simulink library "walk_left_Gait"  (R2024a)
settings: Solver=VariableStepAuto  StartTime=0.0  StopTime=10.0  RelTol=1e-3
undefined symbols (not defined in the file): Lower_limbs, Upper_limbs
libraries: Plane_Movement_walk_left x4
settings Model: Creator=renre  LastModifiedBy=leona

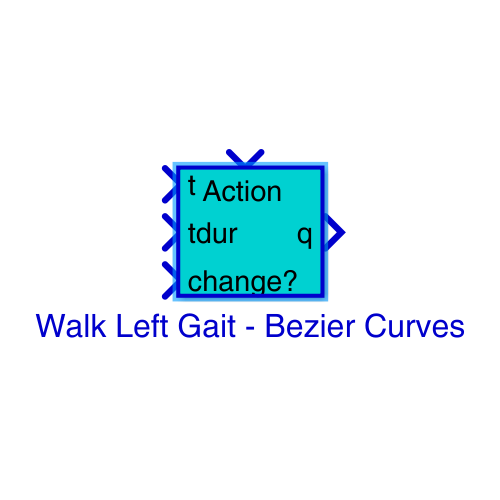
[thumbnail: Simulink's stored preview of the top-level diagram]
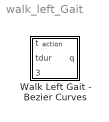
== system walk_left_Gait ==
  Walk Left Gait - Bezier Curves : Subsystem  mask{P0x=-0.02, P0z=-0.08, P1x=-0.035, P1z=-0.06, P2x=0.01, P2z=-0.075, P3x=0.02, P3z=-0.08}
      mask prompts: P0x "Bezier-Point 0 - X"; P0z "Bezier-Point 0 - Z"; P1x "Bezier-Point 1 - X"; P1z "Bezier-Point 1- Z"; P2x "Bezier-Point 2 - X"; P2z "Bezier-Point 2 - Z"; P3x "Bezier-Point 3 - X"; P3z "Bezier-Point 3- Z"

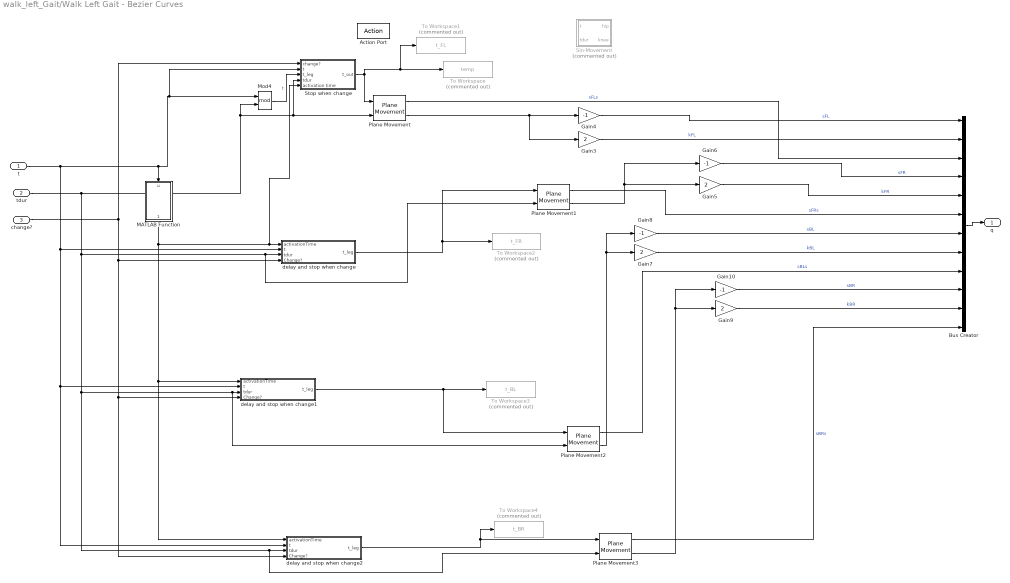
== system walk_left_Gait/Walk Left Gait - Bezier Curves ==
  t : Inport
  tdur : Inport  Port=2
  change? : Inport  Port=3
  Action Port : ActionPort  InitializeStates=reset
  Bus Creator : BusCreator  Inputs=12
  Gain{4,6,8,10} (4 alike) : Gain  Gain=-1
  Gain{3,5,7,9} (4 alike) : Gain  Gain=2
  MATLAB Function : MATLAB Function  TreatAsAtomicUnit=on
  Mod4 : Math  Operator=mod
  Plane Movement{,1..3} (4 alike) : Plane_Movement_walk_left/Plane Movement  SystemSampleTime=-1  VariantActivationTime=update diagram  AllowFlexibleInterface=on  Latency=0  AutoFrameSizeCalculation=off
  Sin-Movement : Subsystem  Commented=on
  Stop when change : Subsystem
  To Workspace : ToWorkspace  Commented=on  VariableName=temp  SaveFormat=Structure With Time  SampleTime=-1
  To Workspace1 : ToWorkspace  Commented=on  VariableName=t_FL  SaveFormat=Structure With Time  SampleTime=-1
  To Workspace2 : ToWorkspace  Commented=on  VariableName=t_FR  SaveFormat=Structure  SampleTime=-1
  To Workspace3 : ToWorkspace  Commented=on  VariableName=t_BL  SaveFormat=Structure  SampleTime=-1
  To Workspace4 : ToWorkspace  Commented=on  VariableName=t_BR  SaveFormat=Structure  SampleTime=-1
  delay and stop when change : Subsystem  mask{delay=0.5}
  delay and stop when change1 : Subsystem  mask{delay=0.25}
  delay and stop when change2 : Subsystem  mask{delay=0.75}
  q : Outport
  wires:
  Bus Creator/1 -> q/1
  Plane Movement/1 -> Bus Creator/3  "sFLs"
  Plane Movement1/1 -> Bus Creator/6  "sFRs"
  Plane Movement/2 -> Gain3/1, Gain4/1
  Plane Movement1/2 -> Gain6/1, Gain5/1
  Plane Movement2/2 -> Gain7/1, Gain8/1
  Plane Movement2/1 -> Bus Creator/9  "sBLs"
  Plane Movement3/2 -> Gain10/1, Gain9/1
  Plane Movement3/1 -> Bus Creator/12  "sBRs"
  Mod4/1 -> Stop when change/3(t_leg)  "t"
  Gain4/1 -> Bus Creator/1  "sFL"
  Gain5/1 -> Bus Creator/5  "kFR"
  Gain6/1 -> Bus Creator/4  "sFR"
  Gain7/1 -> Bus Creator/8  "kBL"
  Gain8/1 -> Bus Creator/7  "sBL"
  Gain9/1 -> Bus Creator/11  "kBR"
  Gain10/1 -> Bus Creator/10  "sBR"
  Gain3/1 -> Bus Creator/2  "kFL"
  Stop when change/1(t_out) -> Plane Movement/1, To Workspace1/1, To Workspace/1
  delay and stop when change2/1(t_leg) -> To Workspace4/1, Plane Movement3/1
  delay and stop when change1/1(t_leg) -> To Workspace3/1, Plane Movement2/1
  delay and stop when change/1(t_leg) -> To Workspace2/1, Plane Movement1/1
  t/1 -> delay and stop when change2/2(t), delay and stop when change1/2(t), delay and stop when change/2(t), Stop when change/2(t), Mod4/1, MATLAB Function/1(u)
  change?/1 -> delay and stop when change2/4(Change?), delay and stop when change1/4(Change?), delay and stop when change/4(Change?), Stop when change/1(change?)
  tdur/1 -> Plane Movement1/2, delay and stop when change/3(tdur), Plane Movement3/2, delay and stop when change2/3(tdur), Plane Movement2/2, delay and stop when change1/3(tdur), Stop when change/4(tdur), Plane Movement/2, Mod4/2
  MATLAB Function/1(activationTime) -> Stop when change/5(activation time), delay and stop when change/1(activationTime), delay and stop when change2/1(activationTime), delay and stop when change1/1(activationTime)

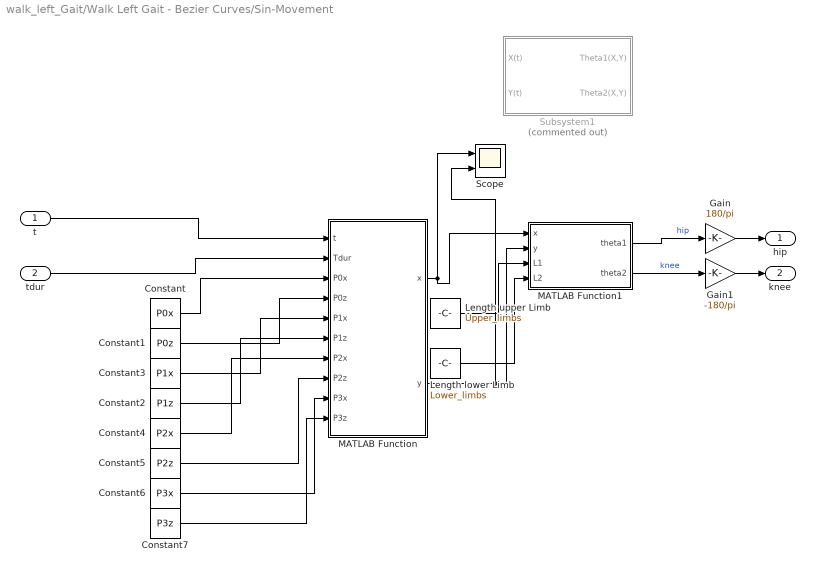
== system walk_left_Gait/Walk Left Gait - Bezier Curves/Sin-Movement ==
  t : Inport
  tdur : Inport  Port=2
  Constant : Constant  Value=P0x
  Constant1 : Constant  Value=P0z
  Constant2 : Constant  Value=P1z
  Constant3 : Constant  Value=P1x
  Constant4 : Constant  Value=P2x
  Constant5 : Constant  Value=P2z
  Constant6 : Constant  Value=P3x
  Constant7 : Constant  Value=P3z
  Gain : Gain  Gain=180/pi
  Gain1 : Gain  Gain=-180/pi
  Length lower Limb : Constant  Value=Lower_limbs
  Length upper Limb : Constant  Value=Upper_limbs
  MATLAB Function : MATLAB Function  TreatAsAtomicUnit=on
  MATLAB Function1 : MATLAB Function  TreatAsAtomicUnit=on
  Scope : Scope  NumInputPorts=2
  Subsystem1 : Subsystem  Commented=on
  hip : Outport
  knee : Outport  Port=2
  wires:
  MATLAB Function/2(y) -> MATLAB Function1/2(y), Scope/2
  MATLAB Function/1(x) -> MATLAB Function1/1(x), Scope/1
  MATLAB Function1/2(theta2) -> Gain1/1  "knee"
  tdur/1 -> MATLAB Function/2(Tdur)
  MATLAB Function1/1(theta1) -> Gain/1  "hip"
  t/1 -> MATLAB Function/1(t)
  Length upper Limb/1 -> MATLAB Function1/3(L1)
  Length lower Limb/1 -> MATLAB Function1/4(L2)
  Gain1/1 -> knee/1
  Gain/1 -> hip/1
  Constant/1 -> MATLAB Function/3(P0x)
  Constant1/1 -> MATLAB Function/4(P0z)
  Constant3/1 -> MATLAB Function/5(P1x)
  Constant2/1 -> MATLAB Function/6(P1z)
  Constant4/1 -> MATLAB Function/7(P2x)
  Constant5/1 -> MATLAB Function/8(P2z)
  Constant6/1 -> MATLAB Function/9(P3x)
  Constant7/1 -> MATLAB Function/10(P3z)

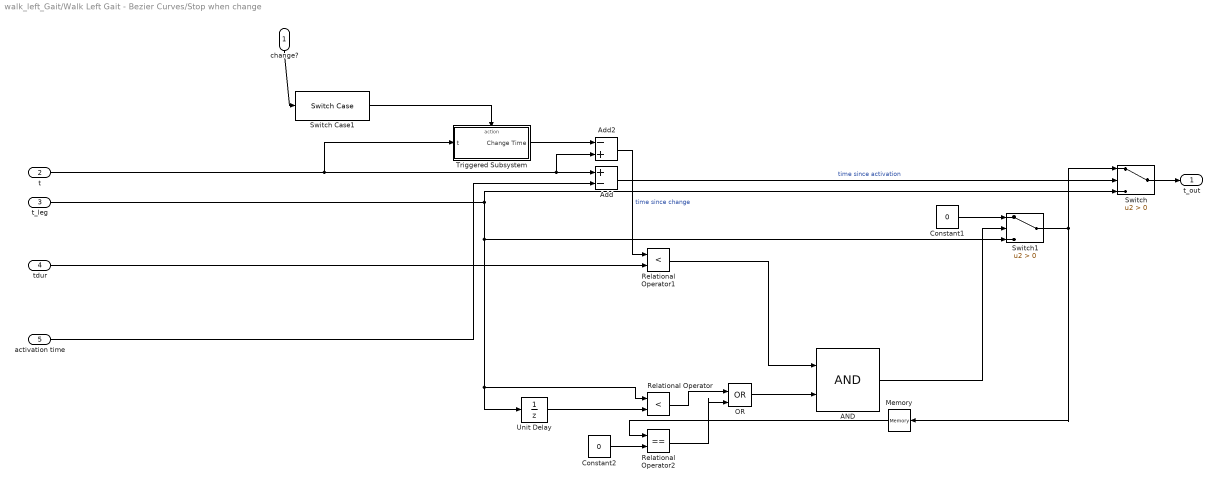
== system walk_left_Gait/Walk Left Gait - Bezier Curves/Stop when change ==
  change? : Inport
  t : Inport  Port=2
  t_leg : Inport  Port=3
  tdur : Inport  Port=4
  activation time : Inport  Port=5
  AND : Logic  IconShape=distinctive  AllPortsSameDT=off  OutDataTypeStr=boolean
  Add : Sum  Inputs=+-
  Add2 : Sum  Inputs=-+
  Constant1 : Constant  Value=0
  Constant2 : Constant  Value=0
  Memory : Memory
  OR : Logic  Operator=OR  IconShape=distinctive  AllPortsSameDT=off  OutDataTypeStr=boolean
  Relational Operator : RelationalOperator  Operator=<  OutDataTypeStr=boolean  RndMeth=Simplest  InputSameDT=off
  Relational Operator1 : RelationalOperator  Operator=<  OutDataTypeStr=boolean  RndMeth=Simplest  InputSameDT=off
  Relational Operator2 : RelationalOperator  Operator===  OutDataTypeStr=boolean  RndMeth=Simplest  InputSameDT=off
  Switch : Switch  Criteria=u2 > Threshold  SaturateOnIntegerOverflow=off  InputSameDT=off
  Switch Case1 : SwitchCase  ShowDefaultCase=off
  Switch1 : Switch  Criteria=u2 > Threshold  SaturateOnIntegerOverflow=off  InputSameDT=off
  Triggered Subsystem : Subsystem  TreatAsAtomicUnit=on
  Unit Delay : UnitDelay  SampleTime=-1  HasFrameUpgradeWarning=on
  t_out : Outport
  wires:
  t_leg/1 -> Switch1/3, Relational Operator/1, Unit Delay/1, Switch/3
  Add2/1 -> Relational Operator1/1  "time since change"
  change?/1 -> Switch Case1/1
  Switch Case1/1 -> Triggered Subsystem/Action
  AND/1 -> Switch1/2
  Unit Delay/1 -> Relational Operator/2
  Switch1/1 -> Memory/1, Switch/1
  Relational Operator1/1 -> AND/1
  Constant2/1 -> Relational Operator2/2
  Triggered Subsystem/1(Change Time) -> Add2/1
  Relational Operator/1 -> OR/1
  tdur/1 -> Relational Operator1/2
  Relational Operator2/1 -> OR/2
  OR/1 -> AND/2
  Constant1/1 -> Switch1/1
  t/1 -> Triggered Subsystem/1(t), Add2/2, Add/1
  Add/1 -> Switch/2  "time since activation"
  Switch/1 -> t_out/1
  activation time/1 -> Add/2
  Memory/1 -> Relational Operator2/1

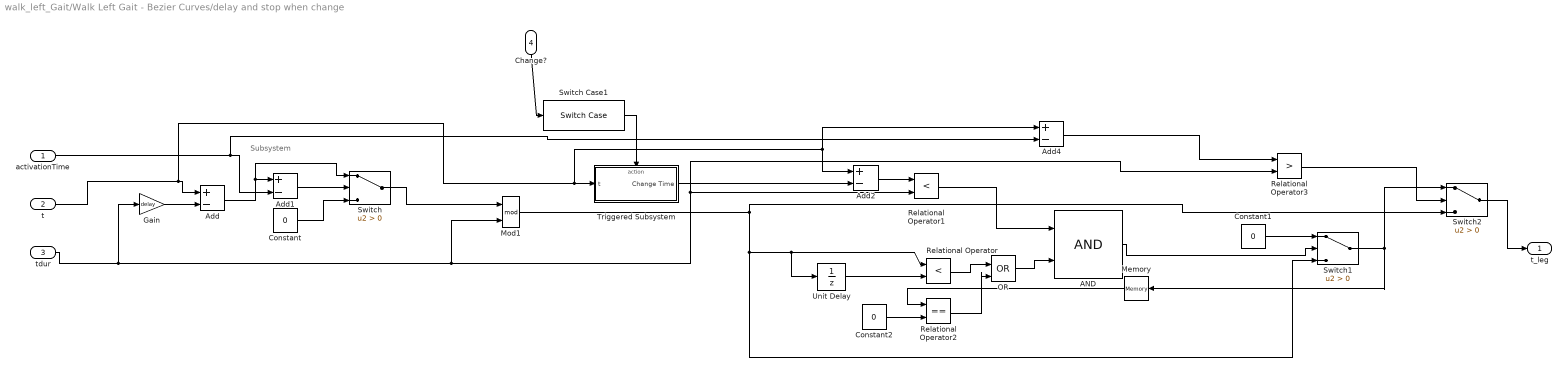
== system walk_left_Gait/Walk Left Gait - Bezier Curves/delay and stop when change ==
  note: Subsystem
  activationTime : Inport
  t : Inport  Port=2
  tdur : Inport  Port=3
  Change? : Inport  Port=4
  AND : Logic  IconShape=distinctive  AllPortsSameDT=off  OutDataTypeStr=boolean
  Add{,1..2,4} (4 alike) : Sum  Inputs=+-
  Constant : Constant  Value=0
  Constant1 : Constant  Value=0
  Constant2 : Constant  Value=0
  Gain : Gain  Gain=delay
  Memory : Memory
  Mod1 : Math  Operator=mod
  OR : Logic  Operator=OR  IconShape=distinctive  AllPortsSameDT=off  OutDataTypeStr=boolean
  Relational Operator : RelationalOperator  Operator=<  OutDataTypeStr=boolean  RndMeth=Simplest  InputSameDT=off
  Relational Operator1 : RelationalOperator  Operator=<  OutDataTypeStr=boolean  RndMeth=Simplest  InputSameDT=off
  Relational Operator2 : RelationalOperator  Operator===  OutDataTypeStr=boolean  RndMeth=Simplest  InputSameDT=off
  Relational Operator3 : RelationalOperator  Operator=>  OutDataTypeStr=boolean  RndMeth=Simplest  InputSameDT=off
  Switch : Switch  Criteria=u2 > Threshold  SaturateOnIntegerOverflow=off  InputSameDT=off
  Switch Case1 : SwitchCase  ShowDefaultCase=off
  Switch1 : Switch  Criteria=u2 > Threshold  SaturateOnIntegerOverflow=off  InputSameDT=off
  Switch2 : Switch  Criteria=u2 > Threshold  SaturateOnIntegerOverflow=off  InputSameDT=off
  Triggered Subsystem : Subsystem  TreatAsAtomicUnit=on
  Unit Delay : UnitDelay  SampleTime=-1  HasFrameUpgradeWarning=on
  t_leg : Outport
  wires:
  Switch/1 -> Mod1/1
  Gain/1 -> Add/2
  t/1 -> Add2/1, Add4/1, Triggered Subsystem/1(t), Add/1
  Constant/1 -> Switch/3
  Add1/1 -> Switch/2
  activationTime/1 -> Add4/2, Add1/2
  Add/1 -> Switch/1, Add1/1
  Switch Case1/1 -> Triggered Subsystem/Action
  Relational Operator1/1 -> AND/1
  Constant1/1 -> Switch1/1
  Relational Operator/1 -> OR/1
  Change?/1 -> Switch Case1/1
  Unit Delay/1 -> Relational Operator/2
  AND/1 -> Switch1/2
  Switch1/1 -> Switch2/1, Memory/1
  Mod1/1 -> Switch2/3, Switch1/3, Unit Delay/1, Relational Operator/1
  Triggered Subsystem/1(Change Time) -> Add2/2
  Add2/1 -> Relational Operator1/1
  Relational Operator2/1 -> OR/2
  Constant2/1 -> Relational Operator2/2
  OR/1 -> AND/2
  Switch2/1 -> t_leg/1
  Relational Operator3/1 -> Switch2/2
  tdur/1 -> Gain/1, Mod1/2, Relational Operator3/2, Relational Operator1/2
  Add4/1 -> Relational Operator3/1
  Memory/1 -> Relational Operator2/1

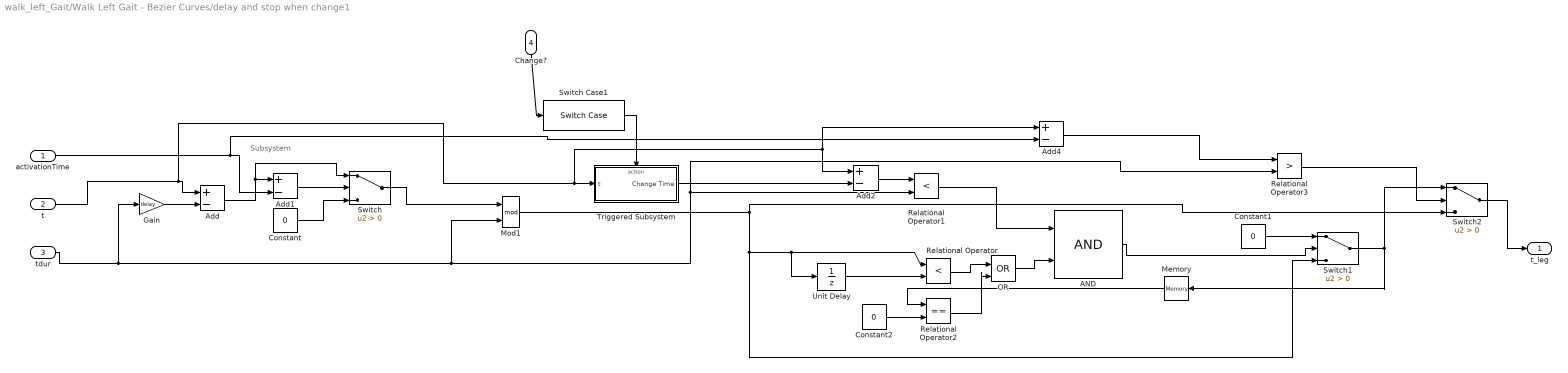
== system walk_left_Gait/Walk Left Gait - Bezier Curves/delay and stop when change1 ==
  note: Subsystem
  activationTime : Inport
  t : Inport  Port=2
  tdur : Inport  Port=3
  Change? : Inport  Port=4
  AND : Logic  IconShape=distinctive  AllPortsSameDT=off  OutDataTypeStr=boolean
  Add{,1..2,4} (4 alike) : Sum  Inputs=+-
  Constant : Constant  Value=0
  Constant1 : Constant  Value=0
  Constant2 : Constant  Value=0
  Gain : Gain  Gain=delay
  Memory : Memory
  Mod1 : Math  Operator=mod
  OR : Logic  Operator=OR  IconShape=distinctive  AllPortsSameDT=off  OutDataTypeStr=boolean
  Relational Operator : RelationalOperator  Operator=<  OutDataTypeStr=boolean  RndMeth=Simplest  InputSameDT=off
  Relational Operator1 : RelationalOperator  Operator=<  OutDataTypeStr=boolean  RndMeth=Simplest  InputSameDT=off
  Relational Operator2 : RelationalOperator  Operator===  OutDataTypeStr=boolean  RndMeth=Simplest  InputSameDT=off
  Relational Operator3 : RelationalOperator  Operator=>  OutDataTypeStr=boolean  RndMeth=Simplest  InputSameDT=off
  Switch : Switch  Criteria=u2 > Threshold  SaturateOnIntegerOverflow=off  InputSameDT=off
  Switch Case1 : SwitchCase  ShowDefaultCase=off
  Switch1 : Switch  Criteria=u2 > Threshold  SaturateOnIntegerOverflow=off  InputSameDT=off
  Switch2 : Switch  Criteria=u2 > Threshold  SaturateOnIntegerOverflow=off  InputSameDT=off
  Triggered Subsystem : Subsystem  TreatAsAtomicUnit=on
  Unit Delay : UnitDelay  SampleTime=-1  HasFrameUpgradeWarning=on
  t_leg : Outport
  wires:
  Switch/1 -> Mod1/1
  Gain/1 -> Add/2
  t/1 -> Add2/1, Add4/1, Triggered Subsystem/1(t), Add/1
  Constant/1 -> Switch/3
  Add1/1 -> Switch/2
  activationTime/1 -> Add4/2, Add1/2
  Add/1 -> Switch/1, Add1/1
  Switch Case1/1 -> Triggered Subsystem/Action
  Relational Operator1/1 -> AND/1
  Constant1/1 -> Switch1/1
  Relational Operator/1 -> OR/1
  Change?/1 -> Switch Case1/1
  Unit Delay/1 -> Relational Operator/2
  AND/1 -> Switch1/2
  Switch1/1 -> Switch2/1, Memory/1
  Mod1/1 -> Switch2/3, Switch1/3, Unit Delay/1, Relational Operator/1
  Triggered Subsystem/1(Change Time) -> Add2/2
  Add2/1 -> Relational Operator1/1
  Relational Operator2/1 -> OR/2
  Constant2/1 -> Relational Operator2/2
  OR/1 -> AND/2
  Switch2/1 -> t_leg/1
  Relational Operator3/1 -> Switch2/2
  tdur/1 -> Gain/1, Mod1/2, Relational Operator3/2, Relational Operator1/2
  Add4/1 -> Relational Operator3/1
  Memory/1 -> Relational Operator2/1

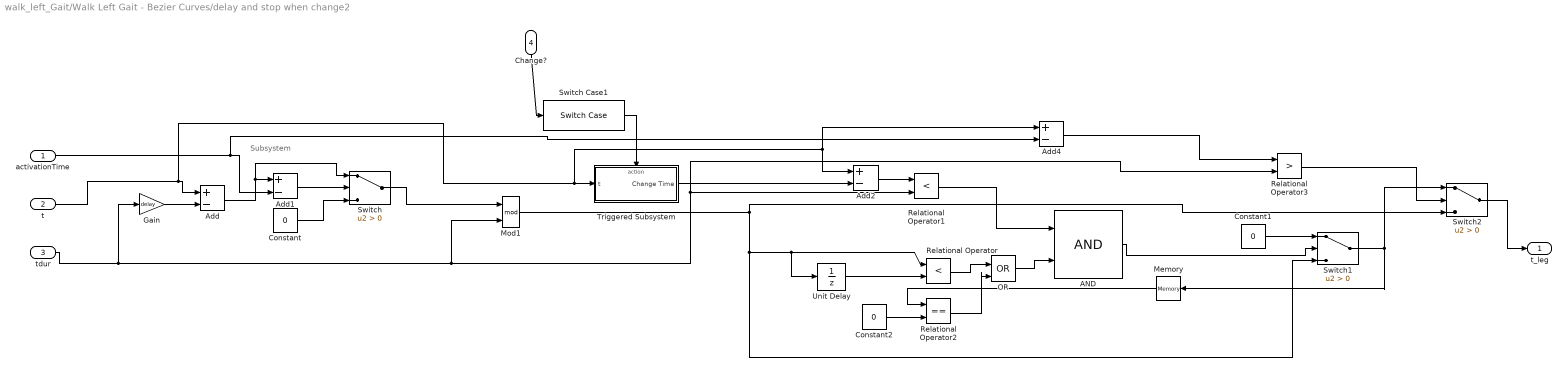
== system walk_left_Gait/Walk Left Gait - Bezier Curves/delay and stop when change2 ==
  note: Subsystem
  activationTime : Inport
  t : Inport  Port=2
  tdur : Inport  Port=3
  Change? : Inport  Port=4
  AND : Logic  IconShape=distinctive  AllPortsSameDT=off  OutDataTypeStr=boolean
  Add{,1..2,4} (4 alike) : Sum  Inputs=+-
  Constant : Constant  Value=0
  Constant1 : Constant  Value=0
  Constant2 : Constant  Value=0
  Gain : Gain  Gain=delay
  Memory : Memory
  Mod1 : Math  Operator=mod
  OR : Logic  Operator=OR  IconShape=distinctive  AllPortsSameDT=off  OutDataTypeStr=boolean
  Relational Operator : RelationalOperator  Operator=<  OutDataTypeStr=boolean  RndMeth=Simplest  InputSameDT=off
  Relational Operator1 : RelationalOperator  Operator=<  OutDataTypeStr=boolean  RndMeth=Simplest  InputSameDT=off
  Relational Operator2 : RelationalOperator  Operator===  OutDataTypeStr=boolean  RndMeth=Simplest  InputSameDT=off
  Relational Operator3 : RelationalOperator  Operator=>  OutDataTypeStr=boolean  RndMeth=Simplest  InputSameDT=off
  Switch : Switch  Criteria=u2 > Threshold  SaturateOnIntegerOverflow=off  InputSameDT=off
  Switch Case1 : SwitchCase  ShowDefaultCase=off
  Switch1 : Switch  Criteria=u2 > Threshold  SaturateOnIntegerOverflow=off  InputSameDT=off
  Switch2 : Switch  Criteria=u2 > Threshold  SaturateOnIntegerOverflow=off  InputSameDT=off
  Triggered Subsystem : Subsystem  TreatAsAtomicUnit=on
  Unit Delay : UnitDelay  SampleTime=-1  HasFrameUpgradeWarning=on
  t_leg : Outport
  wires:
  Switch/1 -> Mod1/1
  Gain/1 -> Add/2
  t/1 -> Add2/1, Add4/1, Triggered Subsystem/1(t), Add/1
  Constant/1 -> Switch/3
  Add1/1 -> Switch/2
  activationTime/1 -> Add4/2, Add1/2
  Add/1 -> Switch/1, Add1/1
  Switch Case1/1 -> Triggered Subsystem/Action
  Relational Operator1/1 -> AND/1
  Constant1/1 -> Switch1/1
  Relational Operator/1 -> OR/1
  Change?/1 -> Switch Case1/1
  Unit Delay/1 -> Relational Operator/2
  AND/1 -> Switch1/2
  Switch1/1 -> Switch2/1, Memory/1
  Mod1/1 -> Switch2/3, Switch1/3, Unit Delay/1, Relational Operator/1
  Triggered Subsystem/1(Change Time) -> Add2/2
  Add2/1 -> Relational Operator1/1
  Relational Operator2/1 -> OR/2
  Constant2/1 -> Relational Operator2/2
  OR/1 -> AND/2
  Switch2/1 -> t_leg/1
  Relational Operator3/1 -> Switch2/2
  tdur/1 -> Gain/1, Mod1/2, Relational Operator3/2, Relational Operator1/2
  Add4/1 -> Relational Operator3/1
  Memory/1 -> Relational Operator2/1

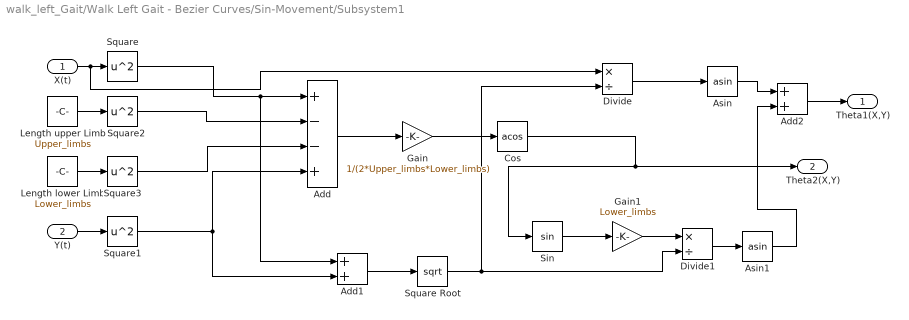
== system walk_left_Gait/Walk Left Gait - Bezier Curves/Sin-Movement/Subsystem1 ==
  X(t) : Inport
  Y(t) : Inport  Port=2
  Add : Sum  Inputs=+--+
  Add1 : Sum
  Add2 : Sum
  Asin : Trigonometry  Operator=asin
  Asin1 : Trigonometry  Operator=asin
  Cos : Trigonometry  Operator=acos
  Divide : Product  Inputs=*/
  Divide1 : Product  Inputs=*/
  Gain : Gain  Gain=1/(2*Upper_limbs*Lower_limbs)
  Gain1 : Gain  Gain=Lower_limbs
  Length lower Limb : Constant  Value=Lower_limbs
  Length upper Limb : Constant  Value=Upper_limbs
  Sin : Trigonometry
  Square{,1..3} (4 alike) : Math  Operator=square
  Square Root : Sqrt
  Theta1(X,Y) : Outport
  Theta2(X,Y) : Outport  Port=2
  wires:
  X(t)/1 -> Divide/1, Square/1
  Y(t)/1 -> Square1/1
  Square/1 -> Add1/1, Add/1
  Length upper Limb/1 -> Square2/1
  Length lower Limb/1 -> Square3/1
  Square2/1 -> Add/2
  Square3/1 -> Add/3
  Square1/1 -> Add1/2, Add/4
  Add/1 -> Gain/1
  Gain/1 -> Cos/1
  Cos/1 -> Theta2(X,Y)/1, Sin/1
  Asin/1 -> Add2/1
  Sin/1 -> Gain1/1
  Add1/1 -> Square Root/1
  Gain1/1 -> Divide1/1
  Square Root/1 -> Divide/2, Divide1/2
  Divide1/1 -> Asin1/1
  Asin1/1 -> Add2/2
  Add2/1 -> Theta1(X,Y)/1
  Divide/1 -> Asin/1

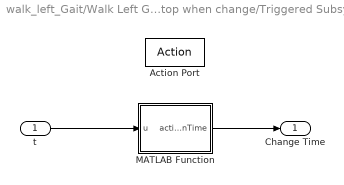
== system walk_left_Gait/Walk Left Gait - Bezier Curves/Stop when change/Triggered Subsystem ==
  t : Inport
  Action Port : ActionPort  InitializeStates=reset
  MATLAB Function : MATLAB Function  TreatAsAtomicUnit=on
  Change Time : Outport
  wires:
  MATLAB Function/1(activationTime) -> Change Time/1
  t/1 -> MATLAB Function/1(u)

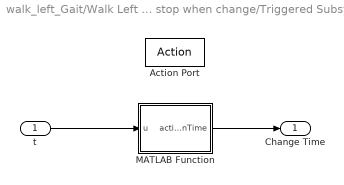
== system walk_left_Gait/Walk Left Gait - Bezier Curves/delay and stop when change/Triggered Subsystem ==
  t : Inport
  Action Port : ActionPort  InitializeStates=reset
  MATLAB Function : MATLAB Function  TreatAsAtomicUnit=on
  Change Time : Outport
  wires:
  MATLAB Function/1(activationTime) -> Change Time/1
  t/1 -> MATLAB Function/1(u)

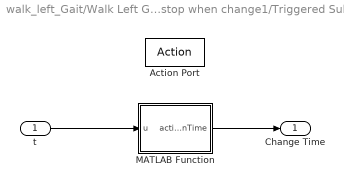
== system walk_left_Gait/Walk Left Gait - Bezier Curves/delay and stop when change1/Triggered Subsystem ==
  t : Inport
  Action Port : ActionPort  InitializeStates=reset
  MATLAB Function : MATLAB Function  TreatAsAtomicUnit=on
  Change Time : Outport
  wires:
  MATLAB Function/1(activationTime) -> Change Time/1
  t/1 -> MATLAB Function/1(u)

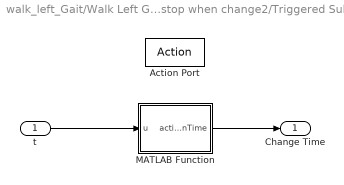
== system walk_left_Gait/Walk Left Gait - Bezier Curves/delay and stop when change2/Triggered Subsystem ==
  t : Inport
  Action Port : ActionPort  InitializeStates=reset
  MATLAB Function : MATLAB Function  TreatAsAtomicUnit=on
  Change Time : Outport
  wires:
  MATLAB Function/1(activationTime) -> Change Time/1
  t/1 -> MATLAB Function/1(u)

== matlab function walk_left_Gait/Walk Left Gait - Bezier Curves/Sin-Movement/MATLAB Function ==
  data: x output; t input; y output; Tdur input; P0x input; P0z input; P1x input; P1z input; P2x input; P2z input; P3x input; P3z input
function [x, y] = bezTrajV2(t, Tdur, P0x,P0z,P1x,P1z,P2x,P2z,P3x,P3z)
t_swing = Tdur/4;
t_support = Tdur*3/4;

P0 = [P0x, P0z];
P1 = [P1x, P1z];
P2 = [P2x, P2z];
P3 = [P3x, P3z];
if t<=t_swing
    Sw = P0*((1-(t/t_swing))^3) + 3*P1*(t/t_swing)*((1-(t/t_swing))^2) + 3*P2*((t/t_swing)^2)*(1-(t/t_swing)) + P3*((t/t_swing)^3);
    
    x = -1*Sw(1);
    y = Sw(2);
else
    x = -1*(P3(1)+(P0(1)-P3(1))/t_support*(t-t_swing));
    y = -0.003*sin((x-P0(1))*pi/(P3(1)-P0(1)))+P0(2);
end
end

== matlab function walk_left_Gait/Walk Left Gait - Bezier Curves/Sin-Movement/MATLAB Function1 ==
  data: x input; theta1 output; y input; L1 input; L2 input; theta2 output
function [theta1, theta2] = ang(x,y,L1,L2)
theta2 = acos((x.^2+y.^2-L1.^2-L2.^2) / (2*L1*L2));
beta = asin((L2*sin(theta2))./((x.^2+y.^2).^0.5));
theta1 = asin(x./((x.^2+y.^2).^0.5)) + beta;
end

== matlab function walk_left_Gait/Walk Left Gait - Bezier Curves/MATLAB Function ==
  data: u input; activationTime output
function activationTime = getActivationTime(u)
    persistent t_start
    if isempty(t_start)
        t_start = u;
    end
    activationTime = t_start;
end

== matlab function walk_left_Gait/Walk Left Gait - Bezier Curves/Stop when change/Triggered Subsystem/MATLAB Function ==
  data: u input; activationTime output
function activationTime = getActivationTime(u)
    persistent t_start
    if isempty(t_start)
        t_start = u;
    end
    activationTime = t_start;
end

== matlab function walk_left_Gait/Walk Left Gait - Bezier Curves/delay and stop when change/Triggered Subsystem/MATLAB Function ==
  data: u input; activationTime output
function activationTime = getActivationTime(u)
    persistent t_start
    if isempty(t_start)
        t_start = u;
    end
    activationTime = t_start;
end

== matlab function walk_left_Gait/Walk Left Gait - Bezier Curves/delay and stop when change1/Triggered Subsystem/MATLAB Function ==
  data: u input; activationTime output
function activationTime = getActivationTime(u)
    persistent t_start
    if isempty(t_start)
        t_start = u;
    end
    activationTime = t_start;
end

== matlab function walk_left_Gait/Walk Left Gait - Bezier Curves/delay and stop when change2/Triggered Subsystem/MATLAB Function ==
  data: u input; activationTime output
function activationTime = getActivationTime(u)
    persistent t_start
    if isempty(t_start)
        t_start = u;
    end
    activationTime = t_start;
end
